simulink model "sampleModel1775_5_sub_sub"  (R2023a)
settings: Solver=VariableStepAuto  StartTime=0.0  StopTime=10.0  RelTol=1e-3
libraries: simulink x4, hdlsllib x1
settings Model: Creator=user1  LastModifiedBy=user1

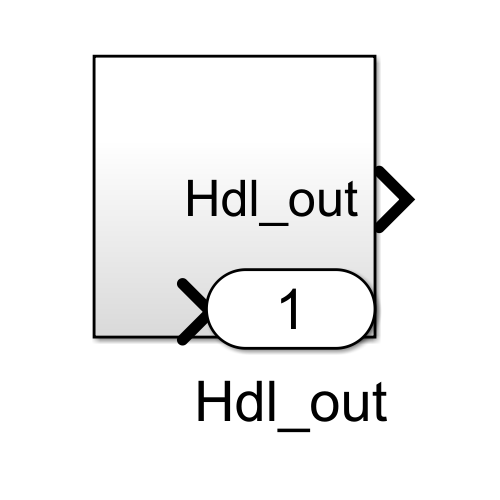
[thumbnail: Simulink's stored preview of the top-level diagram]
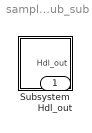
== system sampleModel1775_5_sub_sub ==
  Subsystem : Subsystem
  Hdl_out : Outport  OutDataTypeStr=uint8

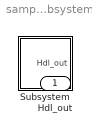
== system sampleModel1775_5_sub_sub/Subsystem ==
  Subsystem : Subsystem
  Hdl_out : Outport  OutDataTypeStr=uint8

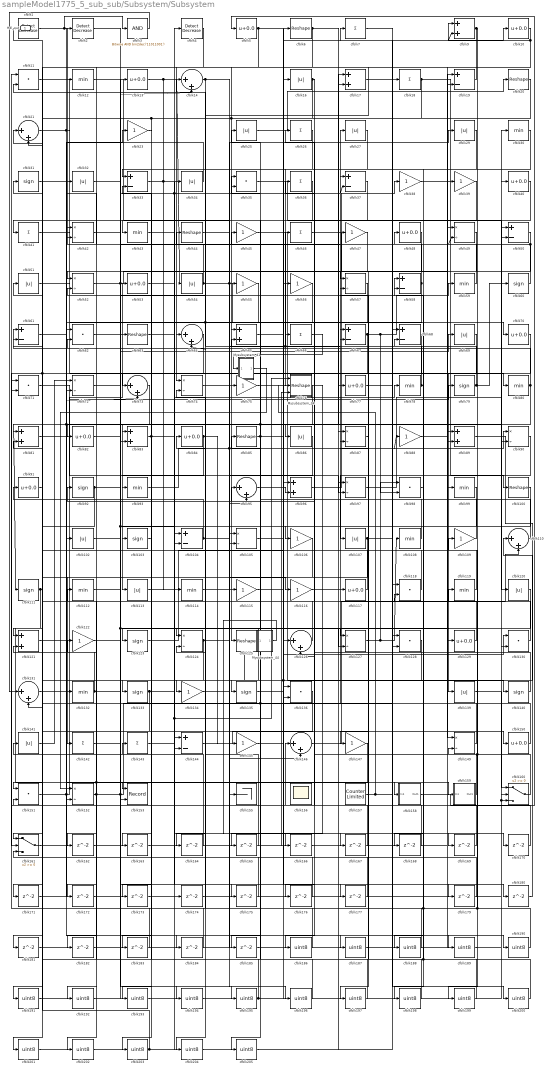
== system sampleModel1775_5_sub_sub/Subsystem/Subsystem ==
  Mysubsystem_34 : Subsystem  TreatAsAtomicUnit=on  RTWFcnName=Mysubsystem_34
      settings: RTWFcnNameOpts=User specified  RTWFileNameOpts=Use function name
  Mysubsystem_41 : Subsystem  TreatAsAtomicUnit=on  RTWFcnName=Mysubsystem_41
      settings: RTWFcnNameOpts=User specified  RTWFileNameOpts=Use function name
  Mysubsystem_44 : Subsystem  TreatAsAtomicUnit=on  RTWFcnName=Mysubsystem_44
      settings: RTWFcnNameOpts=User specified  RTWFileNameOpts=Use function name
  cfblk1 : simulink/Logic and Bit Operations/Detect Decrease  vinit=0.0  OutDataTypeStr=uint8
      settings: LibrarySourceBlock=|
      | hdlsllib/Logic and Bit
      | Operations/Detect
      | Decrease
  cfblk{5,10,13,40,48,53,70,77,82,84,91,117,129,150} (14 alike) : Bias  Bias=0.0  SaturateOnIntegerOverflow=off
  cfblk{6,20,44,63,76,85,100,125} (8 alike) : Reshape
  cfblk{16,25,27,29,32,34,51,54,69,86,102,107,113,120,139,141} (16 alike) : Abs  OutDataTypeStr=uint8  SaturateOnIntegerOverflow=off
  cfblk{31,60,79,92,103,111,123,133,135,140} (10 alike) : Signum
  cfblk{19,33,37,50,58,61,67..68,104,144} (10 alike) : Sum  Inputs=+-  OutDataTypeStr=uint8
  cfblk{42,49,52,57,72,74,87,90,97,105,124,127,149,152} (14 alike) : Product  Inputs=*/  OutDataTypeStr=uint8  RndMeth=Zero  SaturateOnIntegerOverflow=on
  cfblk{23,38..39,45,47,55..56,75,88,106,109,115..116,122,134,145,147} (17 alike) : Gain  OutDataTypeStr=uint8
  cfblk{12,30,43,59,78,80,93,99,108,112,114,119,132} (13 alike) : MinMax  OutDataTypeStr=uint8
  cfblk{11,35,62,71,98,118,128,130,136,151} (10 alike) : DotProduct  OutDataTypeStr=uint8
  cfblk{14,21,64,73,95,110,126,131,146} (9 alike) : Sum  Inputs=|++  OutDataTypeStr=uint8
  cfblk{9,17,65,81,83,89,96,121} (8 alike) : Sum  OutDataTypeStr=uint8
  cfblk{7,18,26,36,41,46,66,142..143} (9 alike) : Sum  Inputs=+  OutDataTypeStr=uint8
  cfblk153 : Record  FileSettingsInternal="{\"entries\":[{\"content\":{\"excelSettings\":{\"content\":{},\"type\":\"Streamout.ExcelSettings\"}},\"type\":\"Streamout.FileSettingStorage\",\"uuid\":\"\"}],\"packageUris\":[\"http:\\/\\/schema.mathworks.com\\/mf0\\/streamout_blocks\\/R2020a\"],\"version\":\"1.0\"}"  Layout=[1 1]  SignalsInternal="{\"entries\":[{\"content\":{\"signals\":[{\"content\":{\"blockPath\":[],\"dimensions\":[1],\"domain\":\"\",\"lineColor\":\"#a2142f\",\"plots\":[1],\"port\":1,\"signalID\":40900,\"signalName\":\"cfblk55\"},\"type\":\"RecordBlkView.Signal\",\"uuid\":\"\"},{\"content\":{\"blockPath\":[],\"dimensions\":[1],\"domain\":\"\",\"lineColor\":\"#139fff\",\"plots\":[1],\"port\":2,\"signalID\":40903,\"signalName\":\"cfblk81\"},\"type\":\"RecordBlkView.Signal\",\"uuid\":\"\"}]},\"type\":\"RecordBlkView.InputSignals\",\"uuid\":\"\"}],\"packageUris\":[\"http:\\/\\/schema.mathworks.com\\/mf0\\/streamout_blocks\\/R2020a\"],\"version\":\"1.0\"}"  VisualizationBindings="{\"xyplotplugin\":{\"info\":[{\"series\":[{\"bindingParametersList\":[{\"parameter\":\"X-Axis\",\"signalID\":40900,\"signalName\":\"cfblk55\"},{\"parameter\":\"Y-Axis\",\"signalID\":40903,\"signalName\":\"cfblk81\"}],\"seriesID\":46410}],\"subplotID\":1}]}}"  CompatibilityTag=XY  st=-1
  cfblk155 : Terminator
  cfblk156 : Scope
      settings: Floating=on
  cfblk157 : hdlsllib/Sources/Counter Limited  uplimit=7  tsamp=-1
  cfblk158 : Subsystem
      settings: LibrarySourceBlock=|
      | hdlsllib/Ports &
      | Subsystems/Subsystem
  cfblk159 : Subsystem
      settings: LibrarySourceBlock=|
      | hdlsllib/Ports &
      | Subsystems/Subsystem
  cfblk160 : Switch  OutDataTypeStr=uint8  SaturateOnIntegerOverflow=off  InputSameDT=off
  cfblk161 : Switch  OutDataTypeStr=uint8  SaturateOnIntegerOverflow=off  InputSameDT=off
  cfblk{162..177,179..185} (23 alike) : Delay  SampleTime=1
  cfblk{186..205} (20 alike) : DataTypeConversion  OutDataTypeStr=uint8  SaturateOnIntegerOverflow=off  RndMeth=Floor
  cfblk2 : simulink/Logic and Bit Operations/Detect Decrease  vinit=0.0  OutDataTypeStr=uint8
      settings: LibrarySourceBlock=|
      | hdlsllib/Logic and Bit
      | Operations/Detect
      | Decrease
  cfblk3 : simulink/Logic and Bit Operations/Bitwise Operator  logicop=AND  UseBitMask=on  BitMask=bin2dec('11011001')  BitMaskRealWorld=Stored Integer
      settings: LibrarySourceBlock=|
      | hdlsllib/Logic and Bit
      | Operations/Bitwise
      | Operator
  cfblk4 : simulink/Logic and Bit Operations/Detect Decrease  vinit=0.0  OutDataTypeStr=uint8
      settings: LibrarySourceBlock=|
      | hdlsllib/Logic and Bit
      | Operations/Detect
      | Decrease
  Hdl_out : Outport  OutDataTypeStr=uint8
  wires:
  Mysubsystem_44/1(Out1) -> cfblk166/1
  Mysubsystem_41/1(Out1) -> cfblk152/1
  cfblk66/1 -> Mysubsystem_41/1(In1)
  Mysubsystem_34/1(Out1) -> cfblk165/1
  cfblk161/1 -> Mysubsystem_34/3(In3)
  cfblk205/1 -> cfblk128/2
  cfblk204/1 -> cfblk128/1
  cfblk203/1 -> cfblk174/1, cfblk151/2
  cfblk202/1 -> cfblk17/2
  cfblk201/1 -> cfblk17/1
  cfblk200/1 -> cfblk161/3, cfblk118/2
  cfblk199/1 -> cfblk87/2
  cfblk198/1 -> cfblk87/1
  cfblk69/1 -> cfblk198/1
  cfblk197/1 -> cfblk85/1
  cfblk87/1 -> cfblk197/1
  cfblk196/1 -> cfblk112/1
  cfblk195/1 -> cfblk130/2, cfblk160/3, cfblk143/1
  cfblk194/1 -> cfblk136/2
  cfblk142/1 -> cfblk194/1
  cfblk193/1 -> cfblk136/1
  cfblk103/1 -> cfblk193/1
  cfblk192/1 -> cfblk63/1
  cfblk136/1 -> cfblk192/1
  cfblk191/1 -> cfblk77/1
  cfblk190/1 -> cfblk68/2, cfblk11/1, cfblk109/1
  cfblk189/1 -> cfblk30/1
  cfblk188/1 -> cfblk84/1
  cfblk30/1 -> cfblk188/1
  cfblk187/1 -> cfblk99/1
  cfblk186/1 -> cfblk141/1
  cfblk99/1 -> cfblk186/1
  cfblk185/1 -> cfblk35/2
  cfblk184/1 -> cfblk144/1
  cfblk122/1 -> cfblk184/1
  cfblk183/1 -> cfblk121/2
  cfblk182/1 -> cfblk95/2
  cfblk47/1 -> cfblk182/1
  cfblk181/1 -> cfblk50/1
  cfblk180/1 -> cfblk110/1
  cfblk82/1 -> cfblk180/1
  cfblk179/1 -> cfblk105/1
  cfblk177/1 -> cfblk124/2
  cfblk176/1 -> cfblk62/1
  cfblk39/1 -> cfblk176/1
  cfblk175/1 -> cfblk131/2
  cfblk174/1 -> cfblk19/2
  cfblk173/1 -> cfblk33/2
  cfblk172/1 -> cfblk160/2
  cfblk64/1 -> cfblk172/1
  cfblk171/1 -> cfblk42/2
  cfblk170/1 -> cfblk71/1
  cfblk169/1 -> cfblk146/1
  cfblk168/1 -> cfblk57/2
  cfblk98/1 -> cfblk168/1
  cfblk167/1 -> cfblk126/2
  cfblk166/1 -> cfblk49/1
  cfblk165/1 -> cfblk74/2
  cfblk164/1 -> cfblk1/1
  cfblk26/1 -> cfblk164/1
  cfblk163/1 -> cfblk96/1
  cfblk100/1 -> cfblk163/1
  cfblk162/1 -> cfblk97/1
  cfblk102/1 -> cfblk129/1
  cfblk62/1 -> cfblk35/1
  cfblk57/1 -> cfblk72/2
  cfblk117/1 -> cfblk61/2
  cfblk74/1 -> cfblk146/2
  cfblk81/1 -> cfblk153/2
  cfblk10/1 -> cfblk9/2, cfblk89/2
  cfblk7/1 -> cfblk68/1
  cfblk131/1 -> cfblk42/1
  cfblk132/1 -> cfblk21/2, cfblk69/1
  cfblk58/1 -> cfblk127/1, cfblk14/1
  cfblk118/1 -> cfblk26/1
  cfblk105/1 -> cfblk10/1
  cfblk128/1 -> cfblk203/1
  cfblk88/1 -> cfblk39/1
  cfblk49/1 -> cfblk147/1
  cfblk85/1 -> cfblk56/1, cfblk25/1
  cfblk80/1 -> cfblk61/1, cfblk134/1
  cfblk6/1 -> cfblk132/1, cfblk89/1
  cfblk68/1 -> cfblk83/1
  cfblk25/1 -> cfblk20/1
  cfblk27/1 -> cfblk33/1
  cfblk44/1 -> cfblk159/1(In1)
  cfblk91/1 -> cfblk51/1
  cfblk129/1 -> cfblk91/1
  cfblk50/1 -> cfblk49/2, cfblk185/1
  cfblk95/1 -> cfblk96/2
  cfblk120/1 -> cfblk144/2
  cfblk40/1 -> cfblk124/1
  cfblk135/1 -> cfblk7/1
  cfblk71/1 -> cfblk126/1
  cfblk23/1 -> cfblk103/1
  cfblk126/1 -> cfblk21/1
  cfblk16/1 -> cfblk106/1, cfblk161/1
  cfblk145/1 -> cfblk130/1
  cfblk63/1 -> cfblk175/1, Mysubsystem_34/1(In1)
  cfblk17/1 -> cfblk200/1
  cfblk56/1 -> cfblk73/1, cfblk64/2
  cfblk41/1 -> cfblk118/1
  cfblk113/1 -> cfblk6/1
  cfblk59/1 -> cfblk12/1
  cfblk97/1 -> cfblk50/2
  cfblk119/1 -> cfblk67/2
  cfblk53/1 -> cfblk90/2
  cfblk108/1 -> cfblk65/2
  cfblk134/1 -> cfblk67/1
  cfblk9/1 -> cfblk121/1, cfblk199/1
  cfblk77/1 -> cfblk190/1
  cfblk33/1 -> cfblk37/2, cfblk169/1, cfblk114/1
  cfblk86/1 -> cfblk105/2
  cfblk32/1 -> cfblk104/2, cfblk179/1
  cfblk65/1 -> Mysubsystem_44/1(In1), cfblk167/1
  cfblk158/1(Out1) -> cfblk5/1
  cfblk42/1 -> cfblk86/1
  cfblk73/1 -> cfblk93/1
  cfblk110/1 -> cfblk45/1
  cfblk157/1 -> Mysubsystem_34/2(In2), cfblk9/1
  cfblk106/1 -> cfblk142/1
  cfblk2/1 -> cfblk127/2, cfblk189/1
  cfblk43/1 -> cfblk97/2
  cfblk115/1 -> cfblk90/1
  cfblk51/1 -> cfblk115/1
  cfblk55/1 -> cfblk153/1
  cfblk133/1 -> cfblk37/1, cfblk181/1
  cfblk159/1(Out1) -> cfblk149/2
  cfblk14/1 -> cfblk116/1, cfblk204/1
  cfblk123/1 -> cfblk16/1
  cfblk61/1 -> cfblk102/1
  cfblk109/1 -> cfblk44/1
  cfblk84/1 -> cfblk113/1, cfblk145/1
  cfblk104/1 -> cfblk55/1, cfblk88/1, cfblk31/1
  cfblk37/1 -> cfblk135/1
  cfblk70/1 -> cfblk71/2
  cfblk93/1 -> cfblk40/1
  cfblk130/1 -> cfblk36/1
  cfblk112/1 -> cfblk195/1
  cfblk160/1 -> cfblk92/1, cfblk119/1
  cfblk5/1 -> cfblk65/1, cfblk177/1
  cfblk60/1 -> cfblk48/1
  cfblk46/1 -> cfblk149/1
  cfblk107/1 -> cfblk170/1, cfblk171/1
  cfblk72/1 -> cfblk13/1
  cfblk21/1 -> cfblk104/1, cfblk73/2
  cfblk152/1 -> cfblk18/1, cfblk14/2, cfblk122/1
  cfblk150/1 -> cfblk95/1, cfblk81/2
  cfblk121/1 -> cfblk79/1
  cfblk11/1 -> cfblk66/1
  cfblk140/1 -> cfblk62/2
  cfblk38/1 -> cfblk19/1
  cfblk13/1 -> cfblk54/1, cfblk34/1
  cfblk35/1 -> cfblk120/1
  cfblk139/1 -> cfblk160/1
  cfblk125/1 -> cfblk123/1, cfblk151/1
  cfblk114/1 -> cfblk75/1
  cfblk3/1 -> cfblk131/1
  cfblk83/1 -> cfblk4/1, cfblk173/1
  cfblk146/1 -> cfblk110/2
  cfblk4/1 -> cfblk64/1
  cfblk12/1 -> cfblk155/1
  cfblk75/1 -> cfblk80/1
  cfblk143/1 -> cfblk78/1
  cfblk151/1 -> cfblk53/1, cfblk23/1
  cfblk54/1 -> cfblk70/1, cfblk196/1, cfblk32/1
  cfblk52/1 -> cfblk57/1, cfblk47/1
  cfblk149/1 -> cfblk117/1
  cfblk31/1 -> cfblk139/1
  cfblk127/1 -> cfblk108/1, cfblk98/1
  cfblk79/1 -> cfblk60/1, cfblk52/2
  cfblk78/1 -> cfblk46/1, cfblk11/2, cfblk58/2
  cfblk111/1 -> cfblk158/1(In1), cfblk191/1
  cfblk36/1 -> cfblk41/1
  cfblk19/1 -> cfblk43/1
  cfblk1/1 -> cfblk83/2, cfblk187/1, cfblk3/1
  cfblk76/1 -> cfblk111/1, cfblk205/1
  cfblk29/1 -> cfblk76/1
  cfblk67/1 -> cfblk81/1, cfblk161/2, cfblk59/1, cfblk98/2
  cfblk147/1 -> cfblk152/2, cfblk162/1
  cfblk124/1 -> cfblk29/1, cfblk202/1
  cfblk141/1 -> cfblk72/1
  cfblk18/1 -> cfblk52/1, cfblk183/1, cfblk100/1
  cfblk34/1 -> cfblk2/1
  cfblk92/1 -> cfblk58/1, cfblk201/1
  cfblk144/1 -> cfblk150/1
  cfblk90/1 -> cfblk107/1
  cfblk48/1 -> cfblk74/1
  cfblk96/1 -> cfblk38/1
  cfblk45/1 -> cfblk140/1
  cfblk116/1 -> cfblk27/1
  cfblk89/1 -> cfblk133/1
  cfblk20/1 -> cfblk125/1, cfblk82/1

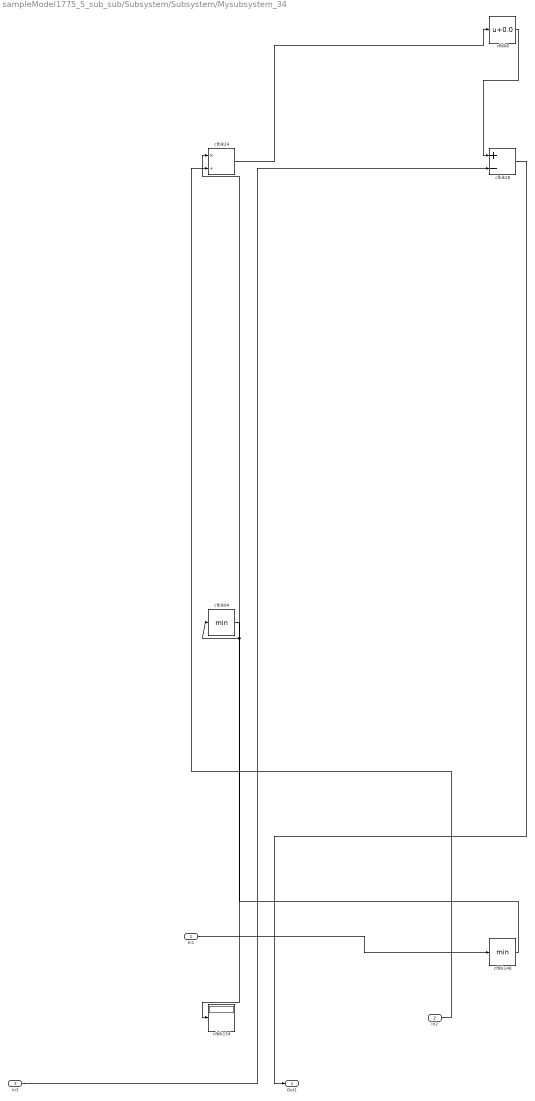
== system sampleModel1775_5_sub_sub/Subsystem/Subsystem/Mysubsystem_34 ==
  In1 : Inport
  In2 : Inport  Port=2
  In3 : Inport  Port=3
  cfblk148 : MinMax
  cfblk154 : Display
  cfblk24 : Product  Inputs=*/  RndMeth=Zero  SaturateOnIntegerOverflow=on
  cfblk28 : Sum  Inputs=+-
  cfblk8 : Bias  Bias=0.0  SaturateOnIntegerOverflow=off
  cfblk94 : MinMax
  Out1 : Outport
  wires:
  cfblk8/1 -> cfblk28/1
  cfblk94/1 -> cfblk154/1
  In3/1 -> cfblk28/2
  In1/1 -> cfblk148/1
  cfblk24/1 -> cfblk8/1
  In2/1 -> cfblk24/2
  cfblk28/1 -> Out1/1
  cfblk148/1 -> cfblk94/1, cfblk24/1

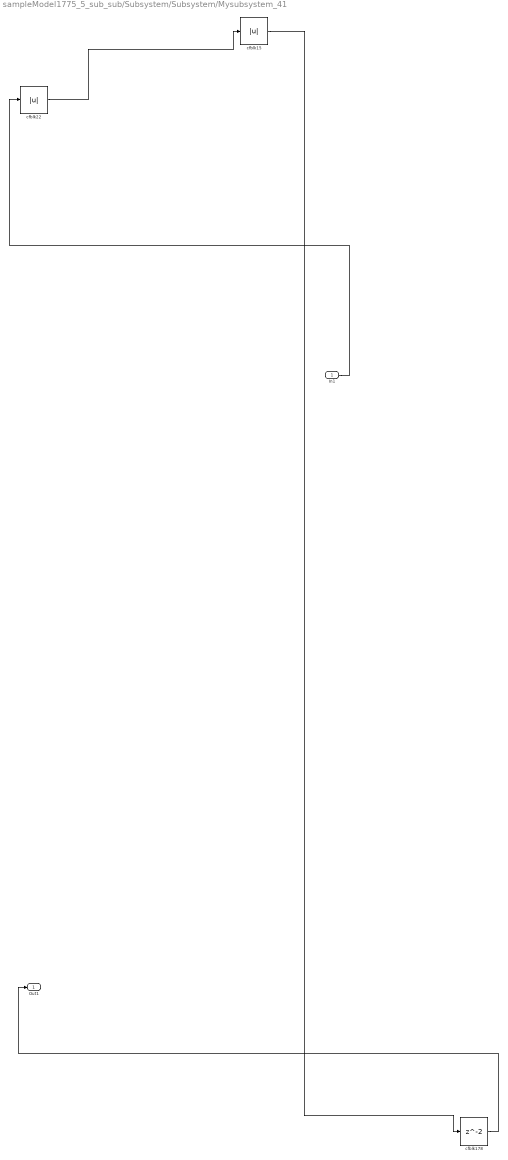
== system sampleModel1775_5_sub_sub/Subsystem/Subsystem/Mysubsystem_41 ==
  In1 : Inport
  cfblk15 : Abs  SaturateOnIntegerOverflow=off
  cfblk178 : Delay  SampleTime=1
  cfblk22 : Abs  SaturateOnIntegerOverflow=off
  Out1 : Outport
  wires:
  cfblk15/1 -> cfblk178/1
  cfblk22/1 -> cfblk15/1
  cfblk178/1 -> Out1/1
  In1/1 -> cfblk22/1

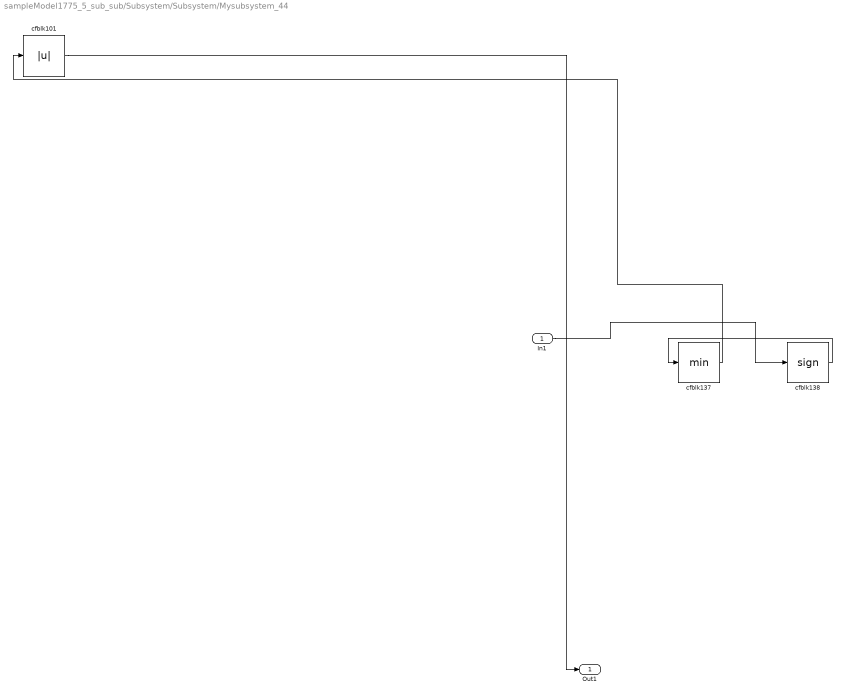
== system sampleModel1775_5_sub_sub/Subsystem/Subsystem/Mysubsystem_44 ==
  In1 : Inport
  cfblk101 : Abs  SaturateOnIntegerOverflow=off
  cfblk137 : MinMax
  cfblk138 : Signum
  Out1 : Outport
  wires:
  cfblk137/1 -> cfblk101/1
  cfblk138/1 -> cfblk137/1
  cfblk101/1 -> Out1/1
  In1/1 -> cfblk138/1

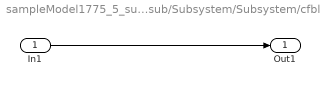
== system sampleModel1775_5_sub_sub/Subsystem/Subsystem/cfblk158 ==
  In1 : Inport
  Out1 : Outport
  wires:
  In1/1 -> Out1/1

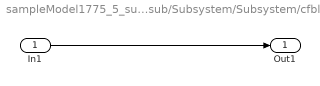
== system sampleModel1775_5_sub_sub/Subsystem/Subsystem/cfblk159 ==
  In1 : Inport
  Out1 : Outport
  wires:
  In1/1 -> Out1/1
